simulink model "Problem_8_Hierarchy"  (R2020a)
settings: Solver=VariableStepAuto  StartTime=0.0  StopTime=10.0  RelTol=1e-3
settings Model: Creator=Admin  LastModifiedBy=Admin

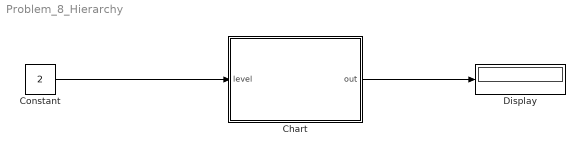
== system Problem_8_Hierarchy ==
  Chart : Stateflow chart  TreatAsAtomicUnit=on
  Constant : Constant  Value=2
  Display : Display
  wires:
  Constant/1 -> Chart/1(level)
  Chart/1(out) -> Display/1

== stateflow chart Problem_8_Hierarchy/Chart ==
  state Run_state
    state stop
      out=cur_st;
    state up
      entry:
      cur_st=cur_st+1;
      out=cur_st;
    state down
      entry:
      cur_st=cur_st-1;
      out=cur_st;
    stop -> stop [order 1] : [level==cur_st]
    (default) -> stop
    stop -> down [order 3] : [cur_st>level]
    stop -> up [order 2] : [cur_st<level]
    up -> stop [order 1] : [cur_st==level]
    down -> stop : [cur_st==level]
    up -> up [order 2] : [cur_st<level]
  state wait
    entry:
    ch=0;
    du:
    ch=ch+1;
  (default) -> Run_state : {cur_st=0;}
  (junction 16) -> stop [order 3]
  (junction 16) -> up [order 1] : [cur_st<level]
  (junction 16) -> down [order 2] : [cur_st>level]
  Run_state -> wait : [cur_st~=level]
  wait -> (junction 16) : [ch==2]
  data: ch local; cur_st local =0; level input; out output
